simulink model "BevraniAGC"  (Simulink 7.8)
settings: Solver=ode45  StartTime=0.0  StopTime=10.0  RelTol=1e-3
libraries: powerlib x1
settings Model: Creator=ywlaw  LastModifiedBy=ywlaw

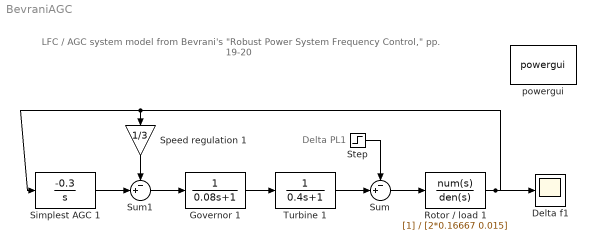
== system BevraniAGC ==
  note: LFC / AGC system model from Bevrani's "Robust Power System Frequency Control," pp. 19-20
  note: Delta PL1
  Delta f1 : Scope
      settings: TimeRange=20
  Governor 1 : TransferFcn  Denominator=[0.08 1]
  Rotor / load 1 : TransferFcn  Denominator=[2*0.16667 0.015]
  Simplest AGC 1 : TransferFcn  Numerator=[-0.3]  Denominator=[1 0]
  Speed regulation 1 : Gain  Gain=1/3
  Step : Step  After=0.02  SampleTime=0  ZeroCross=off
  Sum : Sum  Inputs=-+|
  Sum1 : Sum  Inputs=-+|
  Turbine 1 : TransferFcn  Denominator=[0.4 1]
  powergui : powerlib/powergui  Priority=1  SimulationMode=Continuous  SolverType=Tustin  SampleTime=50e-6  frequency=60  SPID=off  DisableSnubberDevices=off  DisableRonSwitches=off  DisableVfSwitches=off  SwTol=0  Interpol=off  DisplayEquations=off  FunctionMessages=off  frequencyindice=60  Pbase=100e6  ErrMax=1e-4  Iterations=50  UnitsV=kV  UnitsW=MW  echomessages=off  HookPort=off  EnableUseOfTLC=off  x0status=blocks  RestoreLinks=warning  ResistiveCurrentMeasurement=off  Ylog=off  Xlog=on  ShowGrid=off  save=off  variable=ZData  ZoomFFT=off  StartTime=0.0  cycles=1  DisplayStyle=1  FreqAxis=off  MaxFrequency=1000  frequencyindicesteady=1  display=off  methode=off
  wires:
  Turbine 1/1 -> Sum/2
  Governor 1/1 -> Turbine 1/1
  Sum/1 -> Rotor / load 1/1
  Sum1/1 -> Governor 1/1
  Rotor / load 1/1 -> Delta f1/1, Speed regulation 1/1, Simplest AGC 1/1
  Speed regulation 1/1 -> Sum1/1
  Simplest AGC 1/1 -> Sum1/2
  Step/1 -> Sum/1
